simulink model "auntitled"  (R2023a)
settings: Solver=VariableStepAuto  StartTime=0.0  StopTime=10.0  RelTol=1e-3
values from neighbouring files (symbols this model uses):
  A_sn = 1 + 10    (= 11)    [save_student_number.m]    (also in ssn2.m = 18)
  B_sn = 9 + 10    (= 19)    [save_student_number.m]    (also in ssn2.m = 16)
  C_sn = 1 + 10    (= 11)    [save_student_number.m]    (also in ssn2.m = 17)
  D_sn = 7 + 10    (= 17)    [save_student_number.m]    (also in ssn2.m = 15)
  E_sn = 7 + 10    (= 17)    [save_student_number.m]    (also in ssn2.m = 13)
  F_sn = 0 + 10    (= 10)    [save_student_number.m]    (also in ssn2.m)
  G_sn = 6 + 10    (= 16)    [save_student_number.m]    (also in ssn2.m = 19)
  H_sn = 2 + 10    (= 12)    [save_student_number.m]    (also in ssn2.m = 19)
settings Model: Creator=hsait  LastModifiedBy=hsait

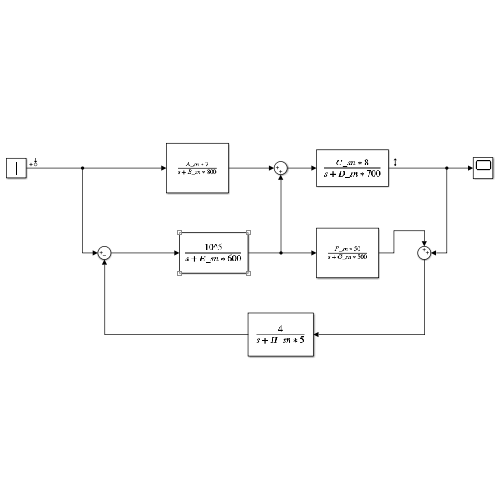
[thumbnail: Simulink's stored preview of the top-level diagram]
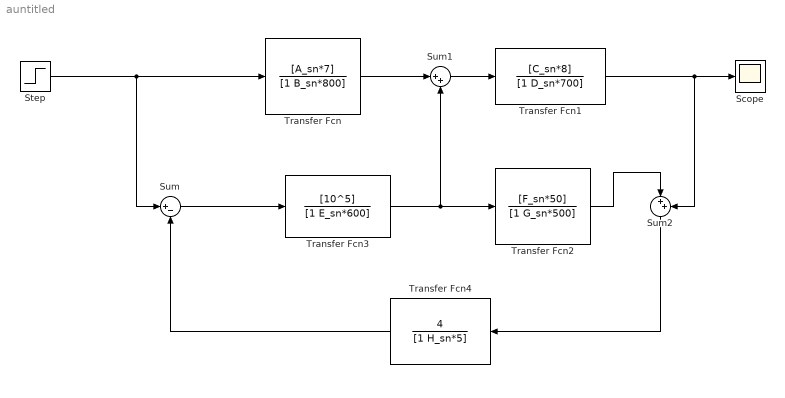
== system auntitled ==
  Scope : Scope
  Step : Step  SampleTime=0
  Sum : Sum  Inputs=|+-
  Sum1 : Sum  Inputs=|++
  Sum2 : Sum  Inputs=|++
  Transfer Fcn : TransferFcn  Numerator=[A_sn*7]  Denominator=[1 B_sn*800]
  Transfer Fcn1 : TransferFcn  Numerator=[C_sn*8]  Denominator=[1 D_sn*700]
  Transfer Fcn2 : TransferFcn  Numerator=[F_sn*50]  Denominator=[1 G_sn*500]
  Transfer Fcn3 : TransferFcn  Numerator=[10^5]  Denominator=[1 E_sn*600]
  Transfer Fcn4 : TransferFcn  Numerator=[4]  Denominator=[1 H_sn*5]
  wires:
  Transfer Fcn/1 -> Sum1/1
  Sum1/1 -> Transfer Fcn1/1
  Transfer Fcn1/1 -> Sum2/2, Scope/1
  Transfer Fcn2/1 -> Sum2/1
  Sum2/1 -> Transfer Fcn4/1
  Transfer Fcn3/1 -> Sum1/2, Transfer Fcn2/1
  Sum/1 -> Transfer Fcn3/1
  Transfer Fcn4/1 -> Sum/2
  Step/1 -> Transfer Fcn/1, Sum/1
